simulink model "DampedMassSpring"  (R2019b)
settings: Solver=ode4  StartTime=0.0  StopTime=10  FixedStep=.01  RelTol=1e-3
values from neighbouring files (symbols this model uses):
  b = zeros(grid_width,grid_height,2)    [BZ_Simulation.m]
undefined symbols (not defined in the file or in its folder): k, m
settings Model: Creator=Nikita Kuznetsov  LastModifiedBy=Nikita Kuznetsov

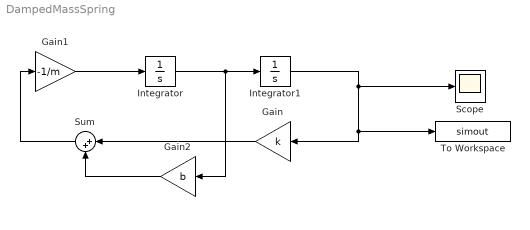
== system DampedMassSpring ==
  Gain : Gain  Gain=k
  Gain1 : Gain  Gain=-1/m
  Gain2 : Gain  Gain=b
  Integrator : Integrator  InitialCondition=.9
  Integrator1 : Integrator  InitialCondition=.6
  Scope : Scope
  Sum : Sum  Inputs=|++
  To Workspace : ToWorkspace  VariableName=simout  SaveFormat=Timeseries  SampleTime=-1
  wires:
  Integrator/1 -> Gain2/1, Integrator1/1
  Integrator1/1 -> To Workspace/1, Gain/1, Scope/1
  Gain2/1 -> Sum/2
  Gain/1 -> Sum/1
  Sum/1 -> Gain1/1
  Gain1/1 -> Integrator/1
